simulink model "Control"  (R2024b)
settings: Solver=FixedStepAuto  StartTime=0.0  StopTime=10.0  RelTol=1e-3
undefined symbols (not defined in the file or in its folder): DiscIntNeverNeededParam
libraries: simulink x3, slpidlib x1
settings Model: DataDictionary=DataDictionary.sldd  Creator=csamak  LastModifiedBy=tsamak
settings OptimizationCC: ZeroExternalMemoryAtStartup=off  ZeroInternalMemoryAtStartup=off  InitFltsAndDblsToZero=on
settings HardwareCC: ProdLongLongMode=on  TargetLongLongMode=on
settings RTWCC: TargetLang=C++  GenerateGPUCode=CUDA
settings GRTTargetCC: TargetLangStandard=C++11 (ISO)  CodeInterfacePackaging=C++ class

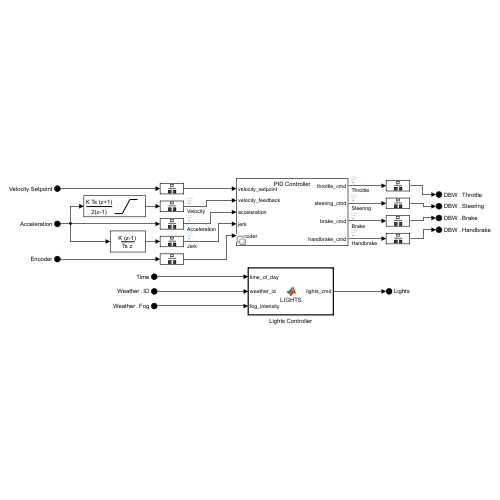
[thumbnail: Simulink's stored preview of the top-level diagram]
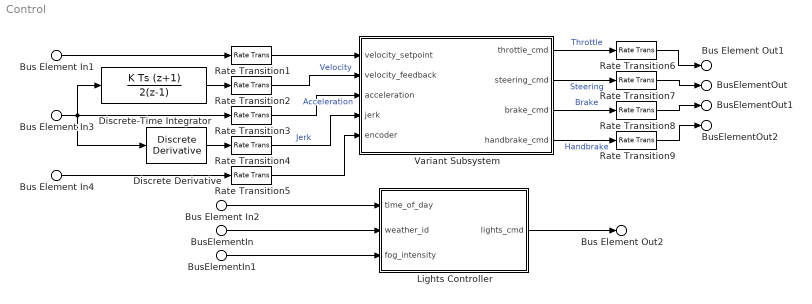
== system Control ==
  Bus Element In1 : Inport  PortName=Velocity Setpoint
  Bus Element In2 : Inport  Port=2  PortName=Time
  BusElementIn : Inport  Port=3  PortName=Weather  Element=ID
  BusElementIn1 : Inport  Port=3  PortName=Weather  Element=Fog
  Bus Element In3 : Inport  Port=4  PortName=Acceleration
  Bus Element In4 : Inport  Port=5  PortName=Encoder
  Discrete Derivative : simulink/Discrete/Discrete Derivative  gainval=1.0  ICPrevScaledInput=0.0  OutMin=[]  OutMax=[]  OutDataType=fixdt(1, 16)  OutScaling=2^-10  DoSatur=off
  Discrete-Time Integrator : DiscreteIntegrator  IntegratorMethod=Integration: Trapezoidal  SampleTime=-1  LimitOutput=on  UpperSaturationLimit=10  LowerSaturationLimit=-10  ICPrevOutput=DiscIntNeverNeededParam  ICPrevScaledInput=DiscIntNeverNeededParam
  Lights Controller : MATLAB Function  TreatAsAtomicUnit=on
  Rate Transition{1..5} (5 alike) : RateTransition  OutPortSampleTime=0.1
  Rate Transition{6..9} (4 alike) : RateTransition  OutPortSampleTime=1
  Variant Subsystem : Subsystem  Variant=on  VariantActivationTime=inherit from Simulink.VariantControl
  Bus Element Out1 : Outport  PortName=DBW  Element=Throttle
  BusElementOut : Outport  PortName=DBW  Element=Steering
  BusElementOut1 : Outport  PortName=DBW  Element=Brake
  BusElementOut2 : Outport  PortName=DBW  Element=Handbrake
  Bus Element Out2 : Outport  Port=2  PortName=Lights
  wires:
  Bus Element In2/1 -> Lights Controller/1(time_of_day)
  Lights Controller/1(lights_cmd) -> Bus Element Out2/1
  BusElementIn/1 -> Lights Controller/2(weather_id)
  BusElementIn1/1 -> Lights Controller/3(fog_intensity)
  Variant Subsystem/1(throttle_cmd) -> Rate Transition6/1  "Throttle"
  Bus Element In3/1 -> Discrete Derivative/1, Rate Transition3/1, Discrete-Time Integrator/1
  Discrete-Time Integrator/1 -> Rate Transition2/1
  Discrete Derivative/1 -> Rate Transition4/1
  Variant Subsystem/2(steering_cmd) -> Rate Transition7/1  "Steering"
  Variant Subsystem/3(brake_cmd) -> Rate Transition8/1  "Brake"
  Variant Subsystem/4(handbrake_cmd) -> Rate Transition9/1  "Handbrake"
  Bus Element In1/1 -> Rate Transition1/1
  Rate Transition2/1 -> Variant Subsystem/2(velocity_feedback)  "Velocity"
  Rate Transition1/1 -> Variant Subsystem/1(velocity_setpoint)
  Rate Transition3/1 -> Variant Subsystem/3(acceleration)  "Acceleration"
  Rate Transition7/1 -> BusElementOut/1
  Rate Transition8/1 -> BusElementOut1/1
  Rate Transition9/1 -> BusElementOut2/1
  Rate Transition6/1 -> Bus Element Out1/1
  Bus Element In4/1 -> Rate Transition5/1
  Rate Transition4/1 -> Variant Subsystem/4(jerk)  "Jerk"
  Rate Transition5/1 -> Variant Subsystem/5(encoder)

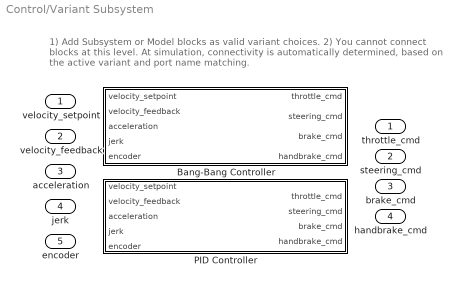
== system Control/Variant Subsystem ==
  note: 1) Add Subsystem or Model blocks as valid variant choices.
      | 2) You cannot connect blocks at this level. At simulation, connectivity is automatically determined, based on the active variant and port name matching.
  velocity_setpoint : Inport
  velocity_feedback : Inport  Port=2
  acceleration : Inport  Port=3
  jerk : Inport  Port=4
  encoder : Inport  Port=5
  Bang-Bang Controller : Subsystem  VariantControl=CONTROLLER==1
  PID Controller : Subsystem  VariantControl=CONTROLLER==2
  throttle_cmd : Outport
  steering_cmd : Outport  Port=2
  brake_cmd : Outport  Port=3
  handbrake_cmd : Outport  Port=4

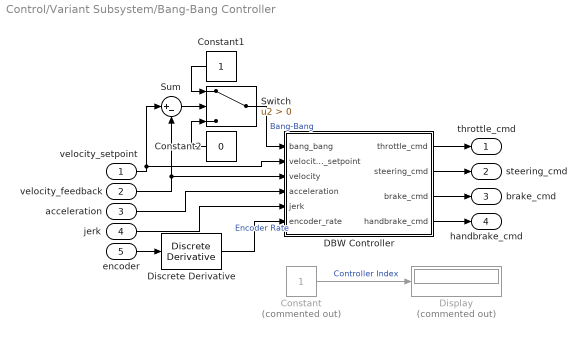
== system Control/Variant Subsystem/Bang-Bang Controller ==
  velocity_setpoint : Inport
  velocity_feedback : Inport  Port=2
  acceleration : Inport  Port=3
  jerk : Inport  Port=4
  encoder : Inport  Port=5
  Constant : Constant  Commented=on
  Constant1 : Constant
  Constant2 : Constant  Value=0
  DBW Controller : MATLAB Function  TreatAsAtomicUnit=on
  Discrete Derivative : simulink/Discrete/Discrete Derivative  gainval=1.0  ICPrevScaledInput=0.0  OutMin=[]  OutMax=[]  OutDataType=fixdt(1, 16)  OutScaling=2^-10  DoSatur=off
  Display : Display  Commented=on
  Sum : Sum  Inputs=|+-
  Switch : Switch  Criteria=u2 > Threshold  SaturateOnIntegerOverflow=off  InputSameDT=off
  throttle_cmd : Outport
  steering_cmd : Outport  Port=2
  brake_cmd : Outport  Port=3
  handbrake_cmd : Outport  Port=4
  wires:
  Constant/1 -> Display/1  "Controller Index"
  Sum/1 -> Switch/2
  Switch/1 -> DBW Controller/1(bang_bang)  "Bang-Bang"
  Constant1/1 -> Switch/1
  Constant2/1 -> Switch/3
  velocity_setpoint/1 -> DBW Controller/2(velocity_setpoint), Sum/1
  acceleration/1 -> DBW Controller/4(acceleration)
  velocity_feedback/1 -> DBW Controller/3(velocity), Sum/2
  DBW Controller/4(handbrake_cmd) -> handbrake_cmd/1
  DBW Controller/1(throttle_cmd) -> throttle_cmd/1
  DBW Controller/3(brake_cmd) -> brake_cmd/1
  DBW Controller/2(steering_cmd) -> steering_cmd/1
  jerk/1 -> DBW Controller/5(jerk)
  Discrete Derivative/1 -> DBW Controller/6(encoder_rate)  "Encoder Rate"
  encoder/1 -> Discrete Derivative/1

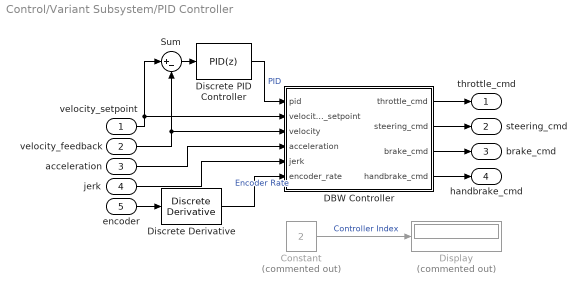
== system Control/Variant Subsystem/PID Controller ==
  velocity_setpoint : Inport
  velocity_feedback : Inport  Port=2
  acceleration : Inport  Port=3
  jerk : Inport  Port=4
  encoder : Inport  Port=5
  Constant : Constant  Commented=on  Value=2
  DBW Controller : MATLAB Function  TreatAsAtomicUnit=on
  Discrete Derivative : simulink/Discrete/Discrete Derivative  gainval=1.0  ICPrevScaledInput=0.0  OutMin=[]  OutMax=[]  OutDataType=fixdt(1, 16)  OutScaling=2^-10  DoSatur=off
  Discrete PID Controller : slpidlib/PID Controller  Controller=PID  Form=Parallel  TimeDomain=Discrete-time  UseExternalTs=off  SampleTime=0.1  IntegratorMethod=Trapezoidal  FilterMethod=Trapezoidal  ControllerParametersSource=internal  P=0.132  I=0.001  UseKiTs=off  D=0.03  UseExternalDerivativeSource=off  N=100  UseFilter=on  TunerSelectOption=Transfer Function Based (PID Tuner App)  InitialConditionSource=internal  InitialConditionForIntegrator=0  InitialConditionForFilter=0  DifferentiatorICPrevScaledInput=0  ExternalReset=none  TrackingMode=off  Kt=1  LimitOutput=on  SatLimitsSource=internal  UpperSaturationLimit=1  LowerSaturationLimit=-1  LinearizeAsGain=off  AntiWindupMode=none  Kb=1  LimitIntegrator=off  UpperIntegratorSaturationLimit=inf  LowerIntegratorSaturationLimit=-inf  POutMin=[]  POutMax=[]  IOutMin=[]  IOutMax=[]  DOutMin=[]  DOutMax=[]  NOutMin=[]  NOutMax=[]  SumOutMin=[]  SumOutMax=[]  SaturationOutMin=[]  SaturationOutMax=[]  PParamMin=[]  PParamMax=[]  IParamMin=[]  IParamMax=[]  DParamMin=[]  DParamMax=[]  NParamMin=[]  NParamMax=[]  KbParamMin=[]  KbParamMax=[]  KtParamMin=[]  KtParamMax=[]  KbOutMin=[]  KbOutMax=[]  KtOutMin=[]  KtOutMax=[]  IntegratorOutMin=[]  IntegratorOutMax=[]  FilterOutMin=[]  FilterOutMax=[]  SumI1OutMin=[]  SumI1OutMax=[]  SumI2OutMin=[]  SumI2OutMax=[]  SumI3OutMin=[]  SumI3OutMax=[]  SumI4OutMin=[]  SumI4OutMax=[]  SumDOutMin=[]  SumDOutMax=[]  DifferentiatorOutMin=[]  DifferentiatorOutMax=[]  FilterDiffOutCoefMin=[]  FilterDiffOutCoefMax=[]  ReciprocalOutMin=[]  ReciprocalOutMax=[]  SumDenOutMin=[]  SumDenOutMax=[]  SumNumOutMin=[]  SumNumOutMax=[]  DivideOutMin=[]  DivideOutMax=[]  UdiffTsProdOutMin=[]  UdiffTsProdOutMax=[]  NTsProdOutMin=[]  NTsProdOutMax=[]  UintegralTsProdOutMin=[]  UintegralTsProdOutMax=[]  UngainTsProdOutMin=[]  UngainTsProdOutMax=[]  ClampingZeroOutDataTypeStr=Inherit: Inherit via back propagation  ClampingZeroOutMin=[]  ClampingZeroOutMax=[]  FilterDenConstantOutDataTypeStr=Inherit: Inherit via back propagation  FilterDenConstantOutMin=[]  FilterDenConstantOutMax=[]  PCopyOutDataTypeStr=Inherit: Inherit via back propagation  PCopyOutMin=[]  PCopyOutMax=[]  NCopyOutDataTypeStr=Inherit: Inherit via back propagation  NCopyOutMin=[]  NCopyOutMax=[]  IntegratorContinuousStateAttributes=''  IntegratorStateMustResolveToSignalObject=off  IntegratorRTWStateStorageClass=Auto  FilterContinuousStateAttributes=''  FilterStateMustResolveToSignalObject=off  FilterRTWStateStorageClass=Auto  ParallelPVariant=InternalParameters  IdealPVariant=Disabled  IVariant=InternalParameters  DVariant=InternalParameters  IntegratorVariant=Discrete  SatVariant=Enabled  AWVariant=Passthrough  PCopyVariant=Disabled  TRVariant=Disabled  FdbkBlocksVariant=Forward  IdealPFdbkVariant=Disabled  SatFdbkVariant=Disabled  DerivativeFilterVariant=TrapezoidalFilter  NVariant=InternalParameters  NCopyVariant=InternalParameters  FilterICVariant=InternalICsFilter  IntegratorICVariant=InternalICs  ExternalResetVariant=Disabled  TRSumVariant=Passthrough  SumFdbkVariant=Disabled  SumVariant=Sum_PID  TsampFilterVariant=InternalTs  TsampNgainVariant=Passthrough  TsampIntegralVariant=Disabled_SignalSpec  ExternalSaturationOutDataTypeStr=Inherit: Same as second input  DerivativeSourceVariant=ErrorSignal  PreIntVariant=InternalPreInt
      settings: LibrarySourceBlock=simulink/Discrete/Discrete PID Controller
  Display : Display  Commented=on
  Sum : Sum  Inputs=|+-
  throttle_cmd : Outport
  steering_cmd : Outport  Port=2
  brake_cmd : Outport  Port=3
  handbrake_cmd : Outport  Port=4
  wires:
  Constant/1 -> Display/1  "Controller Index"
  Sum/1 -> Discrete PID Controller/1
  Discrete PID Controller/1 -> DBW Controller/1(pid)  "PID"
  DBW Controller/4(handbrake_cmd) -> handbrake_cmd/1
  DBW Controller/3(brake_cmd) -> brake_cmd/1
  DBW Controller/2(steering_cmd) -> steering_cmd/1
  DBW Controller/1(throttle_cmd) -> throttle_cmd/1
  acceleration/1 -> DBW Controller/4(acceleration)
  velocity_feedback/1 -> DBW Controller/3(velocity), Sum/2
  velocity_setpoint/1 -> DBW Controller/2(velocity_setpoint), Sum/1
  jerk/1 -> DBW Controller/5(jerk)
  encoder/1 -> Discrete Derivative/1
  Discrete Derivative/1 -> DBW Controller/6(encoder_rate)  "Encoder Rate"

== matlab function Control/Variant Subsystem/PID Controller/DBW Controller ==
  data: pid input; velocity_setpoint input; velocity input; acceleration input; throttle_cmd output; steering_cmd output; brake_cmd output; handbrake_cmd output; jerk input; encoder_rate input
function [throttle_cmd,steering_cmd,brake_cmd,handbrake_cmd] = DBW(pid, velocity_setpoint, velocity, acceleration, jerk, encoder_rate)
    if (velocity_setpoint==0 || encoder_rate<0)
        throttle_cmd=0;
        steering_cmd=0;
        brake_cmd=1;
        handbrake_cmd=0;
    else
        throttle_cmd=max(0, min(0.5, pid));
        brake_cmd=0;
        steering_cmd=0;
        handbrake_cmd=0;
    end

== matlab function Control/Lights Controller ==
  data: time_of_day input; lights_cmd output; weather_id input; fog_intensity input
function lights_cmd  = LIGHTS(time_of_day,weather_id,fog_intensity)
    if (((0 <= time_of_day) && (time_of_day <= 420)) || ((1080 <= time_of_day) && (time_of_day <= 1440))) % Night
        if (weather_id~=1 || weather_id~=2 || (weather_id==0 && fog_intensity ~= 0)) % Foggy night
            lights_cmd = 3; % Vehicle headlights command [0 = Disabled, 1 = Enabled, 2 = Signature Lights, 3 = 1+2]
        else % Clear night
            lights_cmd = 3; % Vehicle headlights command [0 = Disabled, 1 = Enabled, 2 = Signature Lights, 3 = 1+2]
        end
    elseif (weather_id~=1 || weather_id~=2 || (weather_id==0 && fog_intensity ~= 0)) % Foggy day
        lights_cmd = 2; % Vehicle headlights command [0 = Disabled, 1 = Enabled, 2 = Signature Lights, 3 = 1+2]
    else % Clear day
        lights_cmd = 2; % Vehicle headlights command [0 = Disabled, 1 = Enabled, 2 = Signature Lights, 3 = 1+2]
    end

== matlab function Control/Variant Subsystem/Bang-Bang Controller/DBW Controller ==
  data: bang_bang input; velocity_setpoint input; velocity input; acceleration input; throttle_cmd output; steering_cmd output; brake_cmd output; handbrake_cmd output; jerk input; encoder_rate input
function [throttle_cmd,steering_cmd,brake_cmd,handbrake_cmd] = DBW(bang_bang, velocity_setpoint, velocity, acceleration, jerk, encoder_rate)
    if (velocity_setpoint==0 || encoder_rate<0)
        throttle_cmd=0;
        steering_cmd=0;
        brake_cmd=1;
        handbrake_cmd=0;
    else
        throttle_cmd=0.4*bang_bang;
        steering_cmd=0;
        brake_cmd=0.4*(1-bang_bang);
        handbrake_cmd=0;
    end
